simulink model "kalman_w"  (R2023b)
settings: Solver=FixedStepAuto  StartTime=0.0  StopTime=T  FixedStep=dt  RelTol=1e-3
undefined symbols (not defined in the file): A, A_sim_case, B1, B1_sim_case, B2, B2_sim_case, C, C_obs1, C_obs2, C_sim_case, CI, D, D_obs1, D_obs2, D_sim_case, Ko1_kalman_w, Ko2_kalman_w, Kou_kalman_w, T
settings Model: Creator=felipe  LastModifiedBy=felipe

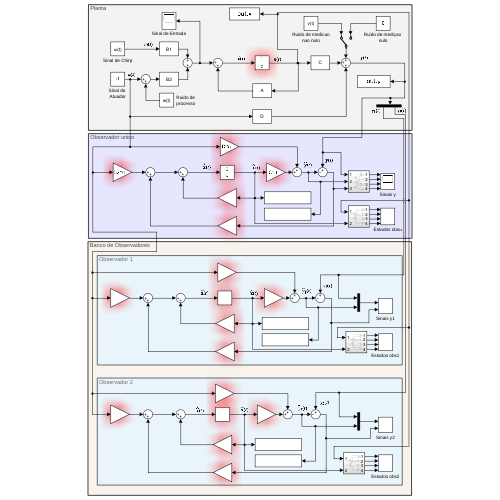
[thumbnail: Simulink's stored preview of the top-level diagram]
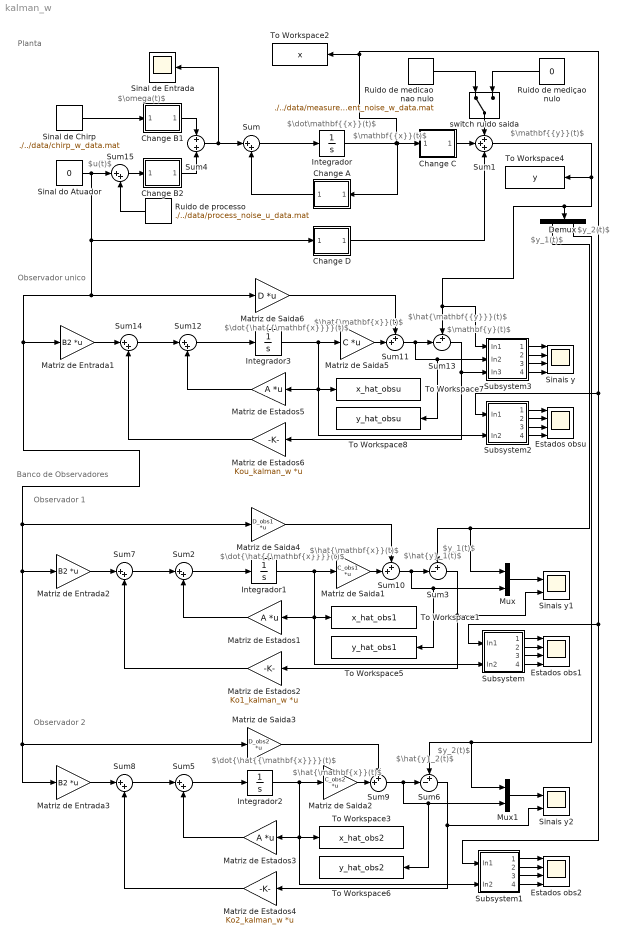
== system kalman_w ==
  note: Observador unico
  note: $\dot{\hat{{\mathbf{x}}}}(t)$
  note: Banco de Observadores
  note: Observador 1
  note: $\omega(t)$
  note: Planta
  note: $\dot\mathbf{{x}}(t)$
  note: $\mathbf{{x}}(t)$
  note: $\mathbf{{y}}(t)$
  note: Observador 2
  note: $y_1(t)$
  note: $y_2(t)$
  note: $\hat{y}_1(t)$
  note: $\hat{\mathbf{x}}(t)$
  note: $\dot{\hat{{\mathbf{x}}}}(t)$
  note: $\hat{y}_2(t)$
  note: $\hat{\mathbf{x}}(t)$
  note: $y_1(t)$
  note: $y_2(t)$
  note: $u(t)$
  note: $\hat{\mathbf{x}}(t)$
  note: $\hat{\mathbf{{y}}}(t)$
  note: $\mathbf{y}(t)$
  note: $\dot{\hat{{\mathbf{x}}}}(t)$
  Change A : Subsystem
      mask Display: disp('A');
  Change B1 : Subsystem
      mask Display: disp('B1');
  Change B2 : Subsystem
      mask Display: disp('B2');
  Change C : Subsystem
      mask Display: disp('C');
  Change D : Subsystem
      mask Display: disp('D');
  Demux : Demux  Outputs=2
  Estados obs1 : Scope  NumInputPorts=4
  Estados obs2 : Scope  NumInputPorts=4
  Estados obsu : Scope  NumInputPorts=4
  Integrador{,1..3} (4 alike) : Integrator  InitialCondition=CI
  Matriz de Entrada1 : Gain  Gain=B2  Multiplication=Matrix(K*u)
  Matriz de Entrada2 : Gain  Gain=B2  Multiplication=Matrix(K*u)
  Matriz de Entrada3 : Gain  Gain=B2  Multiplication=Matrix(K*u)
  Matriz de Estados1 : Gain  Gain=A  Multiplication=Matrix(K*u)
  Matriz de Estados2 : Gain  Gain=Ko1_kalman_w  Multiplication=Matrix(K*u)
  Matriz de Estados3 : Gain  Gain=A  Multiplication=Matrix(K*u)
  Matriz de Estados4 : Gain  Gain=Ko2_kalman_w  Multiplication=Matrix(K*u)
  Matriz de Estados5 : Gain  Gain=A  Multiplication=Matrix(K*u)
  Matriz de Estados6 : Gain  Gain=Kou_kalman_w  Multiplication=Matrix(K*u)
  Matriz de Saida1 : Gain  Gain=C_obs1  Multiplication=Matrix(K*u)
  Matriz de Saida2 : Gain  Gain=C_obs2  Multiplication=Matrix(K*u)
  Matriz de Saida3 : Gain  Gain=D_obs2  Multiplication=Matrix(K*u)
  Matriz de Saida4 : Gain  Gain=D_obs1  Multiplication=Matrix(K*u)
  Matriz de Saida5 : Gain  Gain=C  Multiplication=Matrix(K*u)
  Matriz de Saida6 : Gain  Gain=D  Multiplication=Matrix(K*u)
  Mux : Mux  Inputs=2
  Mux1 : Mux  Inputs=2
  Ruido de processo : FromFile  FileName=./../data/process_noise_u_data.mat  SampleTime=0
      mask Display: disp('w(t)');
  Ruido de medicao nao nulo : FromFile  FileName=./../data/measurement_noise_w_data.mat  SampleTime=0
      mask Display: disp('v(t)');
  Ruido de mediçao nulo : Constant  Value=0
  Sinais y : Scope  NumInputPorts=4
  Sinais y1 : Scope  NumInputPorts=2
  Sinais y2 : Scope  NumInputPorts=2
  Sinal de Chirp : FromFile  FileName=./../data/chirp_w_data.mat  SampleTime=0
      mask Display: disp('ω(t)');
  Sinal de Entrada : Scope
  Sinal do Atuador : Constant  Value=0
  Subsystem : Subsystem
  Subsystem1 : Subsystem
  Subsystem2 : Subsystem
  Subsystem3 : Subsystem
  Sum{,2,5,7..8,12,14..15} (8 alike) : Sum  Inputs=|++
  Sum1 : Sum  Inputs=+++
  Sum10 : Sum  Inputs=++|
  Sum11 : Sum  Inputs=++|
  Sum13 : Sum  Inputs=+-|
  Sum3 : Sum  Inputs=+-|
  Sum4 : Sum
  Sum6 : Sum  Inputs=+-|
  Sum9 : Sum  Inputs=++|
  To Workspace1 : ToWorkspace  VariableName=x_hat_obs1  SampleTime=-1
  To Workspace2 : ToWorkspace  VariableName=x  SampleTime=-1
  To Workspace3 : ToWorkspace  VariableName=x_hat_obs2  SampleTime=-1
  To Workspace4 : ToWorkspace  VariableName=y  SampleTime=-1
  To Workspace5 : ToWorkspace  VariableName=y_hat_obs1  SampleTime=-1
  To Workspace6 : ToWorkspace  VariableName=y_hat_obs2  SampleTime=-1
  To Workspace7 : ToWorkspace  VariableName=x_hat_obsu  SampleTime=-1
  To Workspace8 : ToWorkspace  VariableName=y_hat_obsu  SampleTime=-1
  switch ruido saida : ManualSwitch
  wires:
  Change A/1(v_bm) -> Sum/2
  Sinal de Chirp/1 -> Change B1/1(v_am)
  Change B1/1(v_bm) -> Sum4/1
  switch ruido saida/1 -> Sum1/1
  Ruido de mediçao nulo/1 -> switch ruido saida/2
  Ruido de medicao nao nulo/1 -> switch ruido saida/1
  Sum4/1 -> Sinal de Entrada/1, Sum/1
  Sum3/1 -> Matriz de Estados2/1, Sinais y1/2
  Integrador1/1 -> Matriz de Saida1/1, To Workspace1/1, Subsystem/2(In2), Matriz de Estados1/1
  Sum2/1 -> Integrador1/1
  Matriz de Estados1/1 -> Sum2/2
  Matriz de Estados2/1 -> Sum7/2
  Demux/1 -> Mux/1, Sum3/1
  Integrador2/1 -> Matriz de Saida2/1, To Workspace3/1, Subsystem1/2(In2), Matriz de Estados3/1
  Matriz de Estados3/1 -> Sum5/2
  Sum6/1 -> Matriz de Estados4/1, Sinais y2/2
  Sum5/1 -> Integrador2/1
  Matriz de Saida2/1 -> Sum9/2
  Demux/2 -> Mux1/1, Sum6/1
  Change C/1(v_bm) -> Sum1/2
  Sum7/1 -> Sum2/1
  Matriz de Estados4/1 -> Sum8/2
  Sum8/1 -> Sum5/1
  Matriz de Entrada2/1 -> Sum7/1
  Matriz de Entrada3/1 -> Sum8/1
  Mux/1 -> Sinais y1/1
  Mux1/1 -> Sinais y2/1
  Subsystem/1(Out1) -> Estados obs1/1
  Subsystem/2(Out2) -> Estados obs1/2
  Subsystem/3(Out3) -> Estados obs1/3
  Subsystem/4(Out4) -> Estados obs1/4
  Subsystem1/4(Out4) -> Estados obs2/4
  Subsystem1/3(Out3) -> Estados obs2/3
  Subsystem1/1(Out1) -> Estados obs2/1
  Subsystem1/2(Out2) -> Estados obs2/2
  Sum/1 -> Integrador/1
  Change B2/1(v_bm) -> Sum4/2
  Change D/1(v_bm) -> Sum1/3
  Sum9/1 -> Sum6/2, To Workspace6/1, Mux1/2
  Matriz de Saida3/1 -> Sum9/1
  Matriz de Saida1/1 -> Sum10/2
  Sum10/1 -> To Workspace5/1, Mux/2, Sum3/2
  Matriz de Saida4/1 -> Sum10/1
  Matriz de Entrada1/1 -> Sum14/1
  Matriz de Saida5/1 -> Sum11/2
  Sum14/1 -> Sum12/1
  Subsystem2/1(Out1) -> Estados obsu/1
  Subsystem2/3(Out3) -> Estados obsu/3
  Matriz de Saida6/1 -> Sum11/1
  Integrador3/1 -> Matriz de Saida5/1, To Workspace7/1, Subsystem2/2(In2), Matriz de Estados5/1
  Subsystem2/2(Out2) -> Estados obsu/2
  Sum12/1 -> Integrador3/1
  Subsystem2/4(Out4) -> Estados obsu/4
  Matriz de Estados6/1 -> Sum14/2
  Matriz de Estados5/1 -> Sum12/2
  Sum13/1 -> Matriz de Estados6/1, Subsystem3/3(In3)
  Sum11/1 -> Subsystem3/2(In2), To Workspace8/1, Sum13/2
  Sum1/1 -> To Workspace4/1, Subsystem3/1(In1), Sum13/1, Demux/1
  Sinal do Atuador/1 -> Sum15/1, Change D/1(v_am), Matriz de Saida6/1, Matriz de Entrada1/1, Matriz de Saida4/1, Matriz de Saida3/1, Matriz de Entrada3/1, Matriz de Entrada2/1
  Subsystem3/1(Out1) -> Sinais y/1
  Subsystem3/2(Out2) -> Sinais y/2
  Subsystem3/3(Out3) -> Sinais y/3
  Subsystem3/4(Out4) -> Sinais y/4
  Integrador/1 -> Subsystem2/1(In1), Subsystem/1(In1), Subsystem1/1(In1), To Workspace2/1, Change C/1(v_am), Change A/1(v_am)
  Sum15/1 -> Change B2/1(v_am)
  Ruido de processo/1 -> Sum15/2

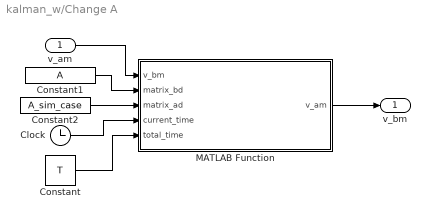
== system kalman_w/Change A ==
  v_am : Inport
  Clock : Clock
  Constant : Constant  Value=T
  Constant1 : Constant  Value=A
  Constant2 : Constant  Value=A_sim_case
  MATLAB Function : MATLAB Function  TreatAsAtomicUnit=on
  v_bm : Outport
  wires:
  Clock/1 -> MATLAB Function/4(current_time)
  MATLAB Function/1(v_am) -> v_bm/1
  v_am/1 -> MATLAB Function/1(v_bm)
  Constant1/1 -> MATLAB Function/2(matrix_bd)
  Constant/1 -> MATLAB Function/5(total_time)
  Constant2/1 -> MATLAB Function/3(matrix_ad)

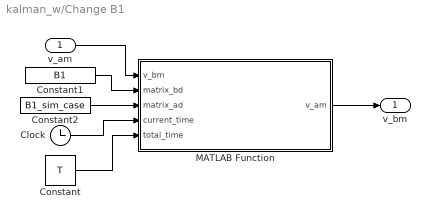
== system kalman_w/Change B1 ==
  v_am : Inport
  Clock : Clock
  Constant : Constant  Value=T
  Constant1 : Constant  Value=B1
  Constant2 : Constant  Value=B1_sim_case
  MATLAB Function : MATLAB Function  TreatAsAtomicUnit=on
  v_bm : Outport
  wires:
  Clock/1 -> MATLAB Function/4(current_time)
  MATLAB Function/1(v_am) -> v_bm/1
  v_am/1 -> MATLAB Function/1(v_bm)
  Constant1/1 -> MATLAB Function/2(matrix_bd)
  Constant/1 -> MATLAB Function/5(total_time)
  Constant2/1 -> MATLAB Function/3(matrix_ad)

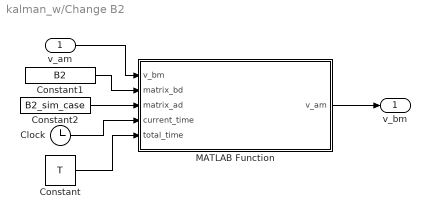
== system kalman_w/Change B2 ==
  v_am : Inport
  Clock : Clock
  Constant : Constant  Value=T
  Constant1 : Constant  Value=B2
  Constant2 : Constant  Value=B2_sim_case
  MATLAB Function : MATLAB Function  TreatAsAtomicUnit=on
  v_bm : Outport
  wires:
  Clock/1 -> MATLAB Function/4(current_time)
  MATLAB Function/1(v_am) -> v_bm/1
  v_am/1 -> MATLAB Function/1(v_bm)
  Constant1/1 -> MATLAB Function/2(matrix_bd)
  Constant/1 -> MATLAB Function/5(total_time)
  Constant2/1 -> MATLAB Function/3(matrix_ad)

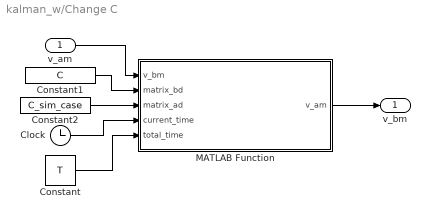
== system kalman_w/Change C ==
  v_am : Inport
  Clock : Clock
  Constant : Constant  Value=T
  Constant1 : Constant  Value=C
  Constant2 : Constant  Value=C_sim_case
  MATLAB Function : MATLAB Function  TreatAsAtomicUnit=on
  v_bm : Outport
  wires:
  Clock/1 -> MATLAB Function/4(current_time)
  MATLAB Function/1(v_am) -> v_bm/1
  v_am/1 -> MATLAB Function/1(v_bm)
  Constant1/1 -> MATLAB Function/2(matrix_bd)
  Constant/1 -> MATLAB Function/5(total_time)
  Constant2/1 -> MATLAB Function/3(matrix_ad)

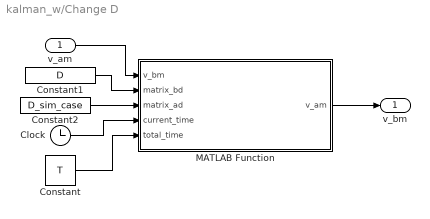
== system kalman_w/Change D ==
  v_am : Inport
  Clock : Clock
  Constant : Constant  Value=T
  Constant1 : Constant  Value=D
  Constant2 : Constant  Value=D_sim_case
  MATLAB Function : MATLAB Function  TreatAsAtomicUnit=on
  v_bm : Outport
  wires:
  Clock/1 -> MATLAB Function/4(current_time)
  MATLAB Function/1(v_am) -> v_bm/1
  v_am/1 -> MATLAB Function/1(v_bm)
  Constant1/1 -> MATLAB Function/2(matrix_bd)
  Constant/1 -> MATLAB Function/5(total_time)
  Constant2/1 -> MATLAB Function/3(matrix_ad)

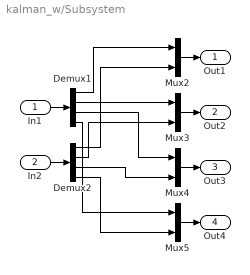
== system kalman_w/Subsystem ==
  In1 : Inport
  In2 : Inport  Port=2
  Demux1 : Demux
  Demux2 : Demux
  Mux{2..5} (4 alike) : Mux  Inputs=2
  Out1 : Outport
  Out2 : Outport  Port=2
  Out3 : Outport  Port=3
  Out4 : Outport  Port=4
  wires:
  Mux5/1 -> Out4/1
  Mux4/1 -> Out3/1
  Mux3/1 -> Out2/1
  Mux2/1 -> Out1/1
  Demux1/3 -> Mux4/1
  Demux2/2 -> Mux3/2
  Demux1/1 -> Mux2/1
  Demux1/2 -> Mux3/1
  In2/1 -> Demux2/1
  Demux2/3 -> Mux4/2
  In1/1 -> Demux1/1
  Demux2/4 -> Mux5/2
  Demux1/4 -> Mux5/1
  Demux2/1 -> Mux2/2

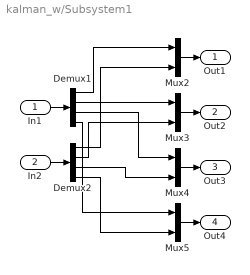
== system kalman_w/Subsystem1 ==
  In1 : Inport
  In2 : Inport  Port=2
  Demux1 : Demux
  Demux2 : Demux
  Mux{2..5} (4 alike) : Mux  Inputs=2
  Out1 : Outport
  Out2 : Outport  Port=2
  Out3 : Outport  Port=3
  Out4 : Outport  Port=4
  wires:
  Mux5/1 -> Out4/1
  Mux4/1 -> Out3/1
  Mux3/1 -> Out2/1
  Mux2/1 -> Out1/1
  Demux1/3 -> Mux4/1
  Demux2/2 -> Mux3/2
  Demux1/1 -> Mux2/1
  Demux1/2 -> Mux3/1
  In2/1 -> Demux2/1
  Demux2/3 -> Mux4/2
  In1/1 -> Demux1/1
  Demux2/4 -> Mux5/2
  Demux1/4 -> Mux5/1
  Demux2/1 -> Mux2/2

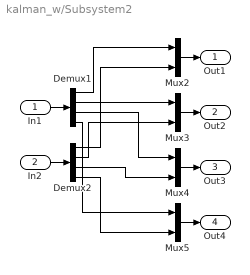
== system kalman_w/Subsystem2 ==
  In1 : Inport
  In2 : Inport  Port=2
  Demux1 : Demux
  Demux2 : Demux
  Mux{2..5} (4 alike) : Mux  Inputs=2
  Out1 : Outport
  Out2 : Outport  Port=2
  Out3 : Outport  Port=3
  Out4 : Outport  Port=4
  wires:
  Mux5/1 -> Out4/1
  Mux4/1 -> Out3/1
  Mux3/1 -> Out2/1
  Mux2/1 -> Out1/1
  Demux1/3 -> Mux4/1
  Demux2/2 -> Mux3/2
  Demux1/1 -> Mux2/1
  Demux1/2 -> Mux3/1
  In2/1 -> Demux2/1
  Demux2/3 -> Mux4/2
  In1/1 -> Demux1/1
  Demux2/4 -> Mux5/2
  Demux1/4 -> Mux5/1
  Demux2/1 -> Mux2/2

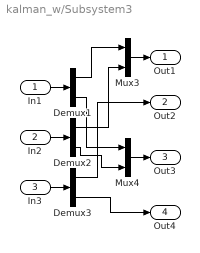
== system kalman_w/Subsystem3 ==
  In1 : Inport
  In2 : Inport  Port=2
  In3 : Inport  Port=3
  Demux1 : Demux  Outputs=2
  Demux2 : Demux  Outputs=2
  Demux3 : Demux  Outputs=2
  Mux3 : Mux  Inputs=2
  Mux4 : Mux  Inputs=2
  Out1 : Outport
  Out2 : Outport  Port=2
  Out3 : Outport  Port=3
  Out4 : Outport  Port=4
  wires:
  Demux1/2 -> Mux4/1
  Demux1/1 -> Mux3/1
  Demux3/1 -> Out2/1
  Demux2/2 -> Mux4/2
  Demux2/1 -> Mux3/2
  Mux4/1 -> Out3/1
  In2/1 -> Demux2/1
  Demux3/2 -> Out4/1
  In1/1 -> Demux1/1
  In3/1 -> Demux3/1
  Mux3/1 -> Out1/1

== matlab function kalman_w/Change B1/MATLAB Function ==
  data: v_bm input; matrix_bd input; matrix_ad input; v_am output; current_time input; total_time input
function v_am = change_matrix(v_bm, matrix_bd, matrix_ad, current_time, total_time)
    if current_time < total_time/2
        v_am = matrix_bd*v_bm;
        return
    end
    v_am = matrix_ad*v_bm;
end

== matlab function kalman_w/Change D/MATLAB Function ==
  data: v_bm input; matrix_bd input; matrix_ad input; v_am output; current_time input; total_time input
function v_am = change_matrix(v_bm, matrix_bd, matrix_ad, current_time, total_time)
    if current_time < total_time/2
        v_am = matrix_bd*v_bm;
        return
    end
    v_am = matrix_ad*v_bm;
end

== matlab function kalman_w/Change A/MATLAB Function ==
  data: v_bm input; matrix_bd input; matrix_ad input; v_am output; current_time input; total_time input
function v_am = change_matrix(v_bm, matrix_bd, matrix_ad, current_time, total_time)
    if current_time < total_time/2
        v_am = matrix_bd*v_bm;
        return
    end
    v_am = matrix_ad*v_bm;
end

== matlab function kalman_w/Change C/MATLAB Function ==
  data: v_bm input; matrix_bd input; matrix_ad input; v_am output; current_time input; total_time input
function v_am = change_matrix(v_bm, matrix_bd, matrix_ad, current_time, total_time)
    if current_time < total_time/2
        v_am = matrix_bd*v_bm;
        return
    end
    v_am = matrix_ad*v_bm;
end

== matlab function kalman_w/Change B2/MATLAB Function ==
  data: v_bm input; matrix_bd input; matrix_ad input; v_am output; current_time input; total_time input
function v_am = change_matrix(v_bm, matrix_bd, matrix_ad, current_time, total_time)
    if current_time < total_time/2
        v_am = matrix_bd*v_bm;
        return
    end
    v_am = matrix_ad*v_bm;
end
